simulink model "RC_calculation"  (R2024b)
settings: Solver=VariableStepAuto  StartTime=0.0  StopTime=50  MaxStep=1e-4  RelTol=1e-3
libraries: spsSeriesRLCBranchLib x2, spsControlledVoltageSourceLib x1, spsGroundLib x1, spsStairGeneratorLib x1, spsVoltageMeasurementLib x1, sps_lib x1
settings Model: SimulationMode=accelerator  Creator=user  LastModifiedBy=user

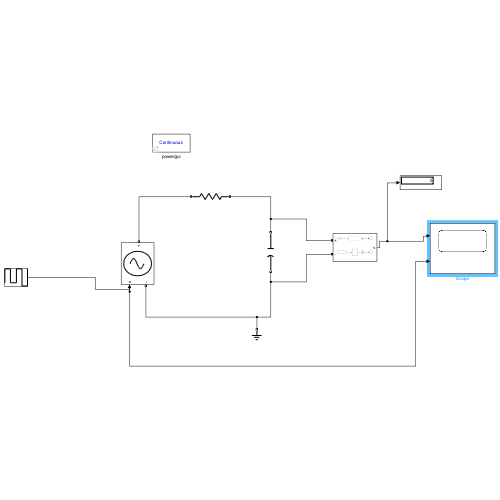
[thumbnail: Simulink's stored preview of the top-level diagram]
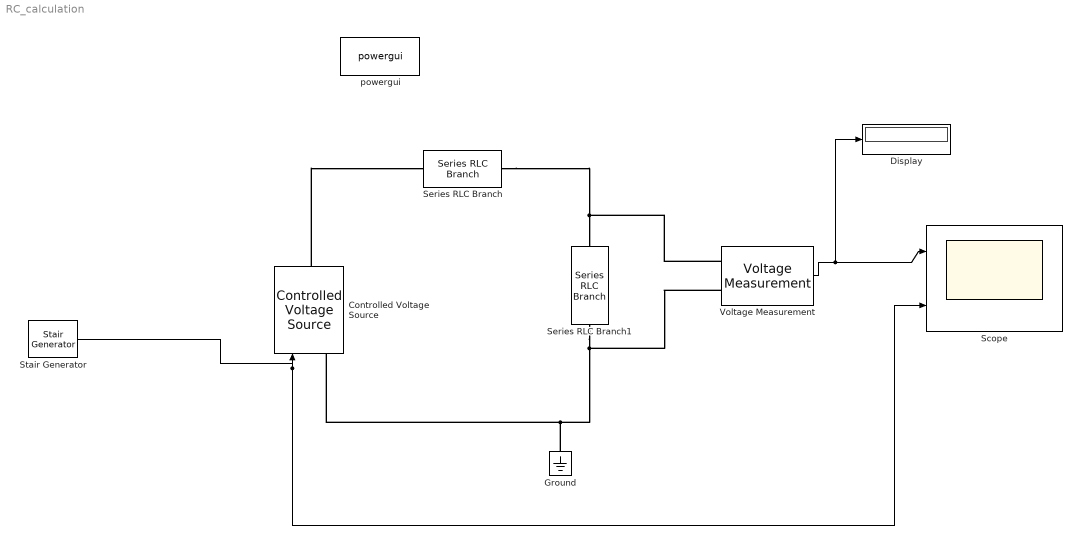
== system RC_calculation ==
  Controlled Voltage Source : spsControlledVoltageSourceLib/Controlled Voltage Source  Initialize=on  Source_Type=DC  Amplitude=5  Phase=0  Frequency=0  Measurements=None
  Display : Display
  Ground : spsGroundLib/Ground  LConnTagsString=a
  Scope : Scope  NumInputPorts=2
  Series RLC Branch : spsSeriesRLCBranchLib/Series RLC Branch  LConnTagsString=__new0  RConnTagsString=__new0  BranchType=R  Resistance=1000  Inductance=1e-3  SetiL0=off  InitialCurrent=0  Capacitance=1e-6  Setx0=off  InitialVoltage=0  Measurements=None
  Series RLC Branch1 : spsSeriesRLCBranchLib/Series RLC Branch  LConnTagsString=__new0  RConnTagsString=__new0  BranchType=C  Resistance=1  Inductance=1e-3  SetiL0=off  InitialCurrent=0  Capacitance=2000e-6  Setx0=on  InitialVoltage=0  Measurements=None
  Stair Generator : spsStairGeneratorLib/Stair Generator  t=[0, 2, 4, 6,8,10]  e=[1, 5,1,5,0,5]  Ts=0
  Voltage Measurement : spsVoltageMeasurementLib/Voltage Measurement  PhasorSimulation=off  OutputType=Complex  PSBequivalent=0
  powergui : sps_lib/powergui  Priority=1  SimulationMode=Continuous  SampleTime=50e-6  frequency=60  Iterations=50  frequencyindice=0  Pbase=100e6  ErrMax=1e-4  UnitsV=kV  UnitsW=MW  buscounter=0  FunctionMessages=off  echomessages=off  EnableUseOfTLC=off  CurrentSourceSwitches=off  DisableSnubberDevices=off  DisableRonSwitches=off  DisableVfSwitches=off  DisplayEquations=off  AutomaticDiscreteSolvers=off  SolverType=Tustin/Backward Euler (TBE)  Interpol=off  ExternalGateDelay=off  methode=off  Ts=100  x0status=blocks  SPID=on  SwTol=0  HookPort=off  NonlinearTolerance=1e-4  nMaxIteration=100  ContinueOnMaxIteration=off  RestoreLinks=warning  ResistiveCurrentMeasurement=off  Frange=[0:2:500]  Ylog=off  Xlog=on  ShowGrid=off  save=off  variable=ZData  structure=0  ZoomFFT=off  StartTime=0.0  cycles=1  DisplayStyle=1  fundamental=60  FreqAxis=off  MaxFrequency=1000  frequencyindicesteady=1  RmsSteady=1  display=off
  wires:
  Voltage Measurement/1 -> Display/1, Scope/1
  Stair Generator/1 -> Scope/2, Controlled Voltage Source/1
  connections:
  Series RLC Branch/RConn1 -- Voltage Measurement/LConn1 -- Series RLC Branch1/LConn1
  Series RLC Branch1/RConn1 -- Ground/LConn1 -- Controlled Voltage Source/LConn1 -- Voltage Measurement/LConn2
  Controlled Voltage Source/RConn1 -- Series RLC Branch/LConn1
